simulink model "sl_groundvehicleDynamics"  (R2025b)
settings: Solver=ode45  StartTime=0.0  StopTime=2000  RelTol=1e-5  EnableMultiTasking=on
InitFcn:
  | mdl_robot;
values from neighbouring files (symbols this model uses):
  A = [1,0,0,dt,0,0;    0,1,0,0,dt,0;    0,0,1,0,0,dt;    0,0,0,1,0,0;    0,0,0,0,1,0;    0,0,0,0,0,1]    [kalman_init.m]    (also in mdl_robot.m = [ 1 0 0 Ts  0  0)
  B = [ Ts   0 ... (first row only)    [mdl_robot.m]
  C = eye(6)    [mdl_robot.m]
  D = zeros(6,2)    [mdl_robot.m]
  initial_state = [robot.X ; robot.Y; robot.Theta; 0; 0; 0]    [mdl_robot.m]
  optimized_waypoints = cuztomized_wp    [mdl_robot.m]
  R = Const_R .* eye(3)    [kalman_init.m]    (also in mdl_robot.m = 0.00316  * R)
undefined symbols (not defined in the file or in its folder): Discrete, obstacles, robot, Time
libraries: simulink x8, mobileRoboticsLib x6, simulink_extras x2, ctrlSharedLib x1, sharedTrackingLibrary x1
settings Model: Creator=sriramn  LastModifiedBy=minhn
settings SolverCC: ZeroCrossAlgorithm=Adaptive  AlgebraicLoopSolver=TrustRegion
settings DataIOCC: LimitDataPoints=on  SaveFormat=Array  ReturnWorkspaceOutputs=off
settings OptimizationCC: ReuseModelBlockBuffer=off  LifeSpan=inf
settings DebuggingCC: SolverPrmCheckMsg=warning  UnconnectedInputMsg=warning  UnconnectedOutputMsg=warning  UnconnectedLineMsg=warning  AllowSymbolicDim=off  SFUnexpectedBacktrackingDiag=warning  SFNoUnconditionalDefaultTransitionDiag=warning  SFExecutionAtInitializationDiag=none  ArithmeticOperatorsInVariantConditions=warning
settings HardwareCC: ProdBitPerPointer=32.0  ProdBitPerSizeT=32.0  ProdBitPerPtrDiffT=32.0  ProdLargestAtomicFloat=None  ProdIntDivRoundTo=Undefined  ProdEndianess=Unspecified  ProdWordSize=32.0  ProdHWDeviceType=32-bit Generic
settings ModelReferenceCC: EnableRefExpFcnMdlSchedulingChecks=on  ModelReferenceMinAlgLoopOccurrences=on  PropagateSignalLabelsOutOfModel=off
settings SFSimCC: SimUseLocalCustomCode=off  CustomCodeUndefinedFunction=UseInterfaceOnly
settings RTWCC: RTWUseLocalCustomCode=off  GPUComputeCapability=3.5
settings CodeAppCC: StateflowObjectComments=on
settings GRTTargetCC: TargetLangStandard=C89/C90 (ANSI)
settings ConfigComp: CovMetricSettings=dw  CovSaveCumulativeToWorkspaceVar=on  CovSaveSingleToWorkspaceVar=on  CovExternalEMLEnable=off  CovSFcnEnable=off
settings SimscapeCC: SimscapeNormalizeSystem=off  SimscapeLogDataHistory=5000  SimscapeLogDecimation=1
settings ConfigurationSet: Description=SimMechanics 2G
settings ExplorerConfigSet: InternalSimMechanicsExplorerSettings="<ExplorerConfiguration><canonicalview>planar_xy</canonicalview><AnimationSetting><BasePlaybackSpeed>1.0</BasePlaybackSpeed><PlaybackSpeedFactor>1.0</PlaybackSpeedFactor></AnimationSetting><TilePanel><TileInfo><Tiles Columns=\"1\" Count=\"1\" Rows=\"1\"><Column Left=\"2\" Weight=\"1\"/><Column Left=\"1628\"/><Row Top=\"2\" Weight=\"1\"/><Row Top=\"1072\"/><Tile Height=\"1\" Width=\"1\" X=\"0\" Y=\"0\"/></Tiles></TileInfo><SceneInfo><SceneViewer><BGColor><R>0.60000002384185791</R><G>0.60000002384185791</G><B>0.60000002384185791</B></BGColor><Camera><Position><X>0.22951840878551699</X><Y>0.32651610611526627</Y><Z>-0.27215421354393321</Z></Position><Center><X>-0.15775714411666431</X><Y>-0.15462825985839526</Y><Z>0.065702552916005602</Z></Center><Up><X>-0.56030137557930915</X><Y>0.72817587161684794</Y><Z>0.39474329445726858</Z></Up><Left>-0.21481383955700509</Left><Right>0.21481383955700509</Right><Bottom>-0.27569784609469139</Bottom><Top>0.27569784609469139</Top></Camera></SceneViewer></SceneInfo></TilePanel></ExplorerConfiguration>"

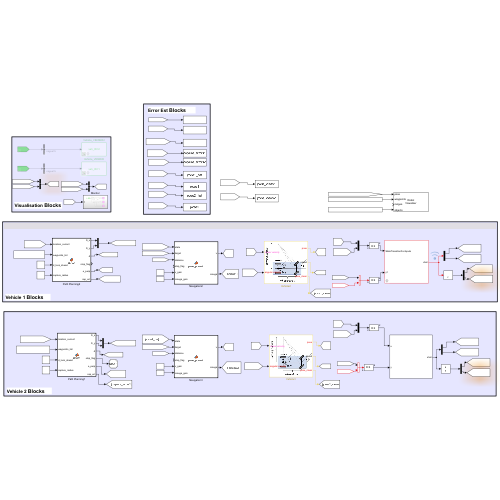
[thumbnail: Simulink's stored preview of the top-level diagram]
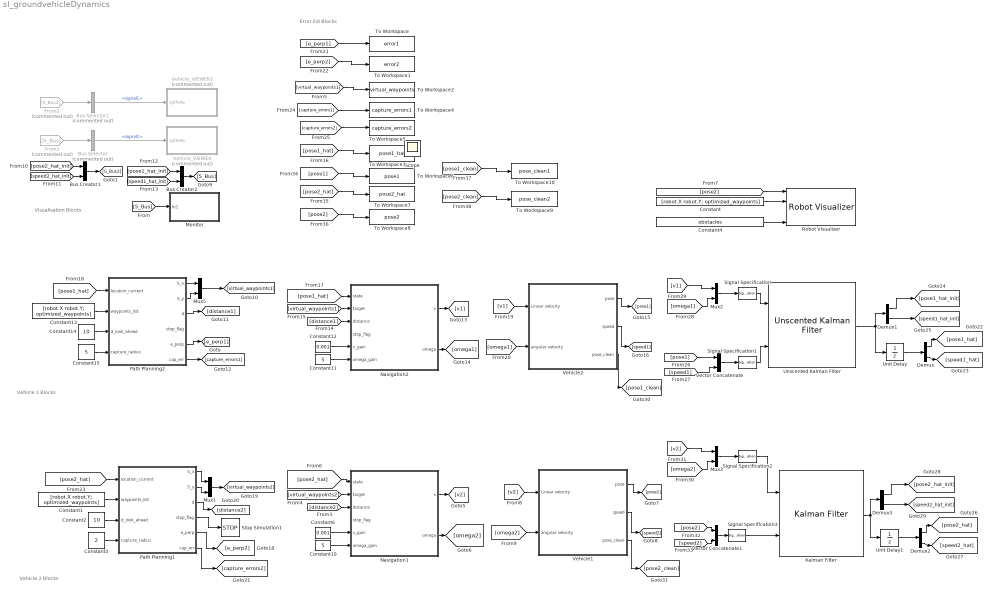
== system sl_groundvehicleDynamics ==
  note: Visualisation Blocks
  note: Vehicle 1 Blocks
  note: Vehicle 2 Blocks
  note: Error Est Blocks
  Bus Creator1 : BusCreator  Inputs=2
  Bus Creator2 : BusCreator  Inputs=2
  Bus Selector : BusSelector  Commented=on  OutputSignals=signal1
  Bus Selector1 : BusSelector  Commented=on  OutputSignals=signal1
  Constant : Constant  Value=[robot.X robot.Y; optimized_waypoints]
  Constant1 : Constant  Value=[robot.X robot.Y; optimized_waypoints]
  Constant10 : Constant  Value=5
  Constant11 : Constant  Value=5
  Constant12 : Constant  Value=0.001
  Constant13 : Constant  Value=[robot.X robot.Y; optimized_waypoints]
  Constant14 : Constant  Value=10
  Constant15 : Constant  Value=5
  Constant2 : Constant  Value=10
  Constant3 : Constant  Value=2
  Constant4 : Constant  Value=obstacles
  Constant6 : Constant  Value=0.001
  Demux{,1..3} (4 alike) : Demux  Outputs=2
  From1 : From  Commented=on  GotoTag=S_Bus
  From2 : From  Commented=on  GotoTag=S_Bus2
  Kalman Filter : ctrlSharedLib/Kalman Filter  TimeDomain=Discrete-Time  UseCurrentEstimator=on  ModelSource=Individual A, B, C, D matrices  ModelSourceVariable=ss(0.95,1,1,0,1)  A=A  B=B  C=C  D=D  NumberOfStates=6  NumberOfInputs=2  NumberOfOutputs=1  InitialEstimateSource=Dialog  X0=initial_state  P0=10  UseK=off  UseGH=off  NumberOfProcessNoiseInputs=1  G=1  TimeInvariantG=on  H=0  TimeInvariantH=on  Q=Q  TimeInvariantQ=on  R=R  TimeInvariantR=on  N=0  TimeInvariantN=on  AddInputPort=on  AddEnablePort=off  OutputEstimatedY=off  OutputP=off  Ts=-1
  Monitor : Subsystem
  Mux{1..3,5} (4 alike) : Mux  Inputs=2
  Navigation1 : MATLAB Function  TreatAsAtomicUnit=on
  Navigation2 : MATLAB Function  TreatAsAtomicUnit=on
  Path Planning1 : MATLAB Function  TreatAsAtomicUnit=on
  Path Planning2 : MATLAB Function  TreatAsAtomicUnit=on
  Robot Visualizer : mobileRoboticsLib/Environments/Robot Visualizer  robotRadius=0.25  mapName=map  showTrajectory=on  hasWaypoints=on  hasLidar=on  sensorOffset=[ 0, 0 ]  scanAngles=[ -pi/4, 0, pi/4 ]  hasObjDetector=on  objDetectorOffset=[ 0, 0 ]  objDetectorAngle=0  objDetectorFOV=pi/4  objDetectorMaxRange=5  objectColors=[ 1, 0, 0; 0, 1, 0; 0, 0, 1 ]  objectMarkers=s
  Signal Specification : SignalSpecification  Dimensions=2
  Signal Specification1 : SignalSpecification  Dimensions=6
  Signal Specification2 : SignalSpecification  Dimensions=2
  Signal Specification3 : SignalSpecification  Dimensions=6
  Stop Simulation1 : Stop
  To Workspace : ToWorkspace  VariableName=error1  SaveFormat=Timeseries  SampleTime=-1
  To Workspace1 : ToWorkspace  VariableName=error2  SaveFormat=Timeseries  SampleTime=-1
  To Workspace10 : ToWorkspace  VariableName=pose_clean1  SaveFormat=Timeseries  SampleTime=-1
  To Workspace2 : ToWorkspace  VariableName=virtual_waypoints  SaveFormat=Timeseries  SampleTime=-1
  To Workspace3 : ToWorkspace  VariableName=pose1_hat  SaveFormat=Timeseries  SampleTime=-1
  To Workspace4 : ToWorkspace  VariableName=capture_errors1  SaveFormat=Timeseries  SampleTime=-1
  To Workspace5 : ToWorkspace  VariableName=capture_errors2  SaveFormat=Timeseries  SampleTime=-1
  To Workspace6 : ToWorkspace  VariableName=pose1  SaveFormat=Timeseries  SampleTime=-1
  To Workspace7 : ToWorkspace  VariableName=pose2_hat  SaveFormat=Timeseries  SampleTime=-1
  To Workspace8 : ToWorkspace  VariableName=pose2  SaveFormat=Timeseries  SampleTime=-1
  To Workspace9 : ToWorkspace  VariableName=pose_clean2  SaveFormat=Timeseries  SampleTime=-1
  Unit Delay : UnitDelay  InitialCondition=[0;0;0;0;0;0]  SampleTime=-1  HasFrameUpgradeWarning=on
  Unit Delay1 : UnitDelay  InitialCondition=[0;0;0;0;0;0]  SampleTime=-1  HasFrameUpgradeWarning=on
  Unscented Kalman Filter : sharedTrackingLibrary/Unscented Kalman Filter  StateTransitionFcn=fState  HasAdditiveProcessNoise=Additive  ProcessNoise=Q  HasTimeVaryingProcessNoise=off  HasStateTransitionFcnExtraArgument=1  InitialState=initial_state  InitialStateCovariance=P0  Alpha=Alpha  Beta=2  Kappa=0  MeasurementFcn1=hMeas  HasMeasurementEnablePort1=off  HasAdditiveMeasurementNoise1=Additive  MeasurementNoise1=R  HasTimeVaryingMeasurementNoise1=off  HasMeasurementFcnExtraArgument1=0  HasMeasurementWrapping1=on  MeasurementFcn2=myMeasurementFcn  HasMeasurementEnablePort2=off  HasAdditiveMeasurementNoise2=Additive  MeasurementNoise2=1  HasTimeVaryingMeasurementNoise2=off  HasMeasurementFcnExtraArgument2=0  HasMeasurementWrapping2=off  MeasurementFcn3=myMeasurementFcn  HasMeasurementEnablePort3=off  HasAdditiveMeasurementNoise3=Additive  MeasurementNoise3=1  HasTimeVaryingMeasurementNoise3=off  HasMeasurementFcnExtraArgument3=0  HasMeasurementWrapping3=off  MeasurementFcn4=myMeasurementFcn  HasMeasurementEnablePort4=off  HasAdditiveMeasurementNoise4=Additive  MeasurementNoise4=1  HasTimeVaryingMeasurementNoise4=off  HasMeasurementFcnExtraArgument4=0  HasMeasurementWrapping4=off  MeasurementFcn5=myMeasurementFcn  HasMeasurementEnablePort5=off  HasAdditiveMeasurementNoise5=Additive  MeasurementNoise5=1  HasTimeVaryingMeasurementNoise5=off  HasMeasurementFcnExtraArgument5=0  HasMeasurementWrapping5=off  EnableMultirate=off  StateTransitionFcnSampleTime=1  MeasurementFcn1SampleTime=1  MeasurementFcn2SampleTime=1  MeasurementFcn3SampleTime=1  MeasurementFcn4SampleTime=1  MeasurementFcn5SampleTime=1  UseCurrentEstimator=on  OutputStateCovariance=off  DataType=double  SampleTime=0.05  NumberOfMeasurements=1
      settings: LibrarySourceBlock=cstblocks/State Estimation/Unscented Kalman Filter
  Vector Concatenate : Concatenate
  Vector Concatenate1 : Concatenate
  Vehicle1 : Subsystem
      mask Display: image('vehicle.jpg');
  Vehicle2 : Subsystem
      mask Display: image('vehicle.jpg');
  Vehicle_VIEWER : Subsystem  Commented=on  mask{wp_mat=optimized_waypoints, veh_ID_num=1, veh_init_xytheta=[robot.X robot.Y robot.Theta], Ts=0.5}
      mask prompts: wp_mat "Waypoint matrix for arena [x_col, y_col] (m)"; veh_ID_num "Vehicle ID number"; veh_init_xytheta "Initial pose [x,y,theta]"; Ts "Sample time for updating animation (secs)"
      mask TypeOptions veh_ID_num: 1 | 2 | 3 | 4
      mask DialogControl Control2 Prompt: Animate simulation of Differential Drive Robot (DDR)
      mask Display: fprintf('veh_ID=%d',veh_ID_num);
  Vehicle_VIEWER2 : Subsystem  Commented=on  mask{wp_mat=optimized_waypoints, veh_ID_num=2, veh_init_xytheta=[robot.X robot.Y robot.Theta], Ts=0.5}
      mask prompts: wp_mat "Waypoint matrix for arena [x_col, y_col] (m)"; veh_ID_num "Vehicle ID number"; veh_init_xytheta "Initial pose [x,y,theta]"; Ts "Sample time for updating animation (secs)"
      mask TypeOptions veh_ID_num: 1 | 2 | 3 | 4
      mask DialogControl Control2 Prompt: Animate simulation of Differential Drive Robot (DDR)
      mask Display: fprintf('veh_ID=%d',veh_ID_num);
  Scope : Scope
      settings: ActiveDisplayYMinimum=0.07  ActiveDisplayYMaximum=0.09
  wires:
  Constant6/1 -> Navigation1/5(v_gain)
  Vehicle1/1(pose) -> [pose2]
  Constant10/1 -> Navigation1/6(omega_gain)
  [distance2] -> Navigation1/3(distance)
  [virtual_waypoints2] -> Navigation1/2(target)
  Navigation1/1(v) -> [v2]
  [pose2_hat] -> Navigation1/1(state)
  Vehicle1/2(speed) -> [speed2]
  [v2] -> Vehicle1/1(Linear velocity)
  [omega2] -> Vehicle1/2(angular velocity)
  [pose1_hat_init] -> Bus Creator2/1
  Bus Creator2/1 -> [S_Bus]
  [speed1_hat_init] -> Bus Creator2/2
  Bus Creator1/1 -> [S_Bus2]
  [pose2_hat_init] -> Bus Creator1/1
  From2/1 -> Bus Selector1/1
  [speed2_hat_init] -> Bus Creator1/2
  [S_Bus] -> Monitor/1(In1)
  Bus Selector1/1 -> Vehicle_VIEWER2/1(xytheta)  "<signal1>"
  Bus Selector/1 -> Vehicle_VIEWER/1(xytheta)  "<signal1>"
  From1/1 -> Bus Selector/1
  Constant14/1 -> Path Planning2/3(d_look_ahead)
  Navigation2/2(omega) -> [omega1]
  Constant15/1 -> Path Planning2/4(capture_radius)
  Vehicle2/1(pose) -> [pose1]
  Path Planning2/1(S_x) -> Mux5/1
  Mux5/1 -> [virtual_waypoints1]
  [pose1_hat] -> Path Planning2/1(location_current)
  Constant11/1 -> Navigation2/6(omega_gain)
  Constant13/1 -> Path Planning2/2(waypoints_list)
  Path Planning2/2(S_y) -> Mux5/2
  [distance1] -> Navigation2/3(distance)
  [v1] -> Vehicle2/1(Linear velocity)
  Constant12/1 -> Navigation2/5(v_gain)
  [omega1] -> Vehicle2/2(angular velocity)
  Path Planning2/3(d) -> [distance1]
  [pose1_hat] -> Navigation2/1(state)
  [virtual_waypoints1] -> Navigation2/2(target)
  Vehicle2/2(speed) -> [speed1]
  Navigation2/1(v) -> [v1]
  Path Planning2/5(e_perp) -> [e_perp1]
  [e_perp2] -> To Workspace1/1
  [pose2_hat] -> Path Planning1/1(location_current)
  Constant2/1 -> Path Planning1/3(d_look_ahead)
  Path Planning1/5(e_perp) -> [e_perp2]
  Path Planning1/3(d) -> [distance2]
  Constant1/1 -> Path Planning1/2(waypoints_list)
  Constant3/1 -> Path Planning1/4(capture_radius)
  Path Planning1/2(S_y) -> Mux1/2
  Mux1/1 -> [virtual_waypoints2]
  Path Planning1/1(S_x) -> Mux1/1
  [e_perp1] -> To Workspace/1
  [virtual_waypoints1] -> To Workspace2/1
  [pose1_hat] -> To Workspace3/1
  Path Planning2/6(cap_err) -> [capture_errors1]
  [capture_errors1] -> To Workspace4/1
  Path Planning1/6(cap_err) -> [capture_errors2]
  [capture_errors2] -> To Workspace5/1
  Mux2/1 -> Signal Specification/1
  [omega1] -> Mux2/2
  Demux/1 -> [pose1_hat]
  Signal Specification/1 -> Unscented Kalman Filter/1
  Unscented Kalman Filter/1 -> Unit Delay/1, Demux1/1
  Signal Specification1/1 -> Unscented Kalman Filter/2
  [v1] -> Mux2/1
  Demux/2 -> [speed1_hat]
  Unit Delay/1 -> Demux/1
  [pose1] -> Vector Concatenate/1
  Demux1/2 -> [speed1_hat_init]
  Demux1/1 -> [pose1_hat_init]
  [speed1] -> Vector Concatenate/2
  Vector Concatenate/1 -> Signal Specification1/1
  [v2] -> Mux3/1
  Signal Specification2/1 -> Kalman Filter/1
  [omega2] -> Mux3/2
  Mux3/1 -> Signal Specification2/1
  Vector Concatenate1/1 -> Signal Specification3/1
  [speed2] -> Vector Concatenate1/2
  [pose2] -> Vector Concatenate1/1
  Signal Specification3/1 -> Kalman Filter/2
  Demux3/1 -> [pose2_hat_init]
  Unit Delay1/1 -> Demux2/1
  Kalman Filter/1 -> Demux3/1, Unit Delay1/1
  Demux2/1 -> [pose2_hat]
  Demux2/2 -> [speed2_hat]
  Demux3/2 -> [speed2_hat_init]
  Navigation1/2(omega) -> [omega2]
  [pose1] -> To Workspace6/1
  [pose2_hat] -> To Workspace7/1
  [pose2] -> To Workspace8/1
  [pose1_clean] -> To Workspace10/1
  Vehicle2/3(pose_clean) -> [pose1_clean]
  [pose2_clean] -> To Workspace9/1
  Vehicle1/3(pose_clean) -> [pose2_clean]
  Path Planning1/4(stop_flag) -> Stop Simulation1/1
  Constant/1 -> Robot Visualizer/2
  [pose2] -> Robot Visualizer/1
  Constant4/1 -> Robot Visualizer/4

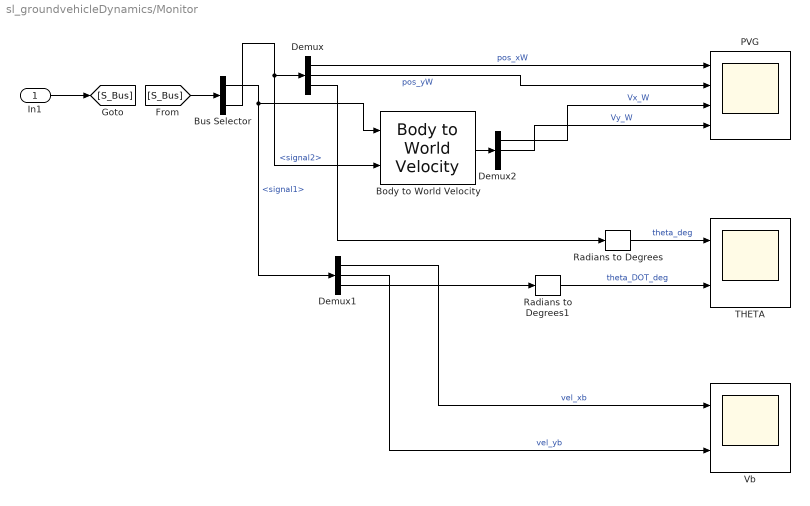
== system sl_groundvehicleDynamics/Monitor ==
  In1 : Inport
  Body to World Velocity : mobileRoboticsLib/Utilities/Body to World Velocity
      settings: SourceProductName=Mobile Robotics Simulation Toolbox
  Bus Selector : BusSelector  OutputSignals=signal1,signal2
  Demux : Demux  Outputs=3
  Demux1 : Demux  Outputs=3
  Demux2 : Demux  Outputs=3
  PVG : Scope  NumInputPorts=4
      settings: ActiveDisplayYMinimum=-3.02358  ActiveDisplayYMaximum=27.35477
  Radians to Degrees : simulink_extras/Transformations/Radians to Degrees
  Radians to Degrees1 : simulink_extras/Transformations/Radians to Degrees
  THETA : Scope  NumInputPorts=2
      settings: ActiveDisplayYMinimum=-8.72937  ActiveDisplayYMaximum=60.06611  DataLoggingVariableName=ScopeData2
  Vb : Scope  NumInputPorts=2
      settings: ActiveDisplayYMinimum=0.05577  ActiveDisplayYMaximum=0.8929
  wires:
  In1/1 -> [S_Bus]
  [S_Bus] -> Bus Selector/1
  Demux/1 -> PVG/1  "pos_xW"
  Demux/2 -> PVG/2  "pos_yW"
  Radians to Degrees1/1 -> THETA/2  "theta_DOT_deg"
  Radians to Degrees/1 -> THETA/1  "theta_deg"
  Demux1/3 -> Radians to Degrees1/1
  Demux/3 -> Radians to Degrees/1
  Bus Selector/1 -> Demux1/1, Body to World Velocity/1  "<signal1>"
  Body to World Velocity/1 -> Demux2/1
  Demux2/1 -> PVG/3  "Vx_W"
  Demux2/2 -> PVG/4  "Vy_W"
  Demux1/1 -> Vb/1  "vel_xb"
  Demux1/2 -> Vb/2  "vel_yb"
  Bus Selector/2 -> Body to World Velocity/2, Demux/1  "<signal2>"

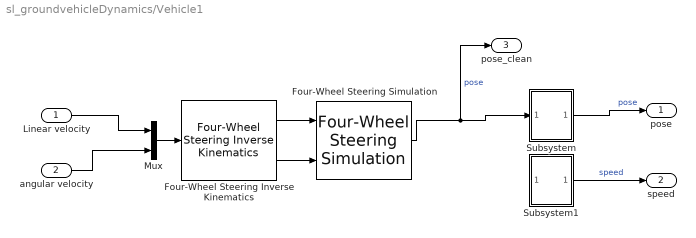
== system sl_groundvehicleDynamics/Vehicle1 ==
  Linear velocity : Inport
  angular velocity : Inport  Port=2
  Four-Wheel Steering Inverse Kinematics : mobileRoboticsLib/Kinematic Models/Four-Wheel Steering/Four-Wheel Steering Inverse Kinematics  wheelRadius=0.1  frontWheelDist=0.25  rearWheelDist=0.25  ikMode=Front Steering
      settings: SourceProductName=Mobile Robotics Simulation Toolbox
  Four-Wheel Steering Simulation : mobileRoboticsLib/Kinematic Models/Four-Wheel Steering/Four-Wheel Steering Simulation  wheelRadius=0.1  frontWheelDist=0.25  rearWheelDist=0.25  initX=robot.X  initY=robot.Y  initAngle=robot.Theta  Ts=0.05
      settings: SourceProductName=Mobile Robotics Simulation Toolbox
  Mux : Mux  Inputs=2
  Subsystem : Subsystem
  Subsystem1 : Subsystem
  pose : Outport  VectorParamsAs1DForOutWhenUnconnected=off
  speed : Outport  Port=2
  pose_clean : Outport  Port=3  VectorParamsAs1DForOutWhenUnconnected=off
  wires:
  angular velocity/1 -> Mux/2
  Linear velocity/1 -> Mux/1
  Mux/1 -> Four-Wheel Steering Inverse Kinematics/1
  Four-Wheel Steering Simulation/1 -> pose_clean/1, Subsystem/1(In1)  "pose"
  ? -> Subsystem1/1(In1)  "speed"
  Four-Wheel Steering Inverse Kinematics/1 -> Four-Wheel Steering Simulation/1
  Four-Wheel Steering Inverse Kinematics/2 -> Four-Wheel Steering Simulation/2
  Subsystem/1(pose) -> pose/1  "pose"
  Subsystem1/1(speed) -> speed/1  "speed"

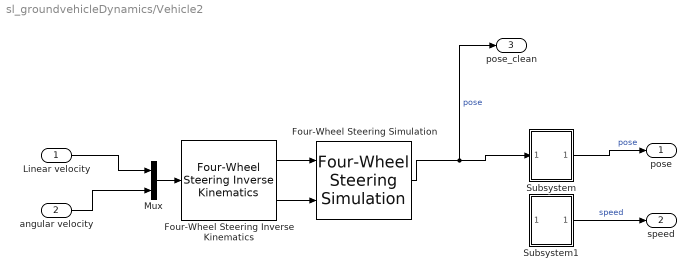
== system sl_groundvehicleDynamics/Vehicle2 ==
  Linear velocity : Inport
  angular velocity : Inport  Port=2
  Four-Wheel Steering Inverse Kinematics : mobileRoboticsLib/Kinematic Models/Four-Wheel Steering/Four-Wheel Steering Inverse Kinematics  wheelRadius=0.1  frontWheelDist=0.25  rearWheelDist=0.25  ikMode=Front Steering
      settings: SourceProductName=Mobile Robotics Simulation Toolbox
  Four-Wheel Steering Simulation : mobileRoboticsLib/Kinematic Models/Four-Wheel Steering/Four-Wheel Steering Simulation  wheelRadius=0.1  frontWheelDist=0.25  rearWheelDist=0.25  initX=robot.X  initY=robot.Y  initAngle=robot.Theta  Ts=0.05
      settings: SourceProductName=Mobile Robotics Simulation Toolbox
  Mux : Mux  Inputs=2
  Subsystem : Subsystem
  Subsystem1 : Subsystem
  pose : Outport  VectorParamsAs1DForOutWhenUnconnected=off
  speed : Outport  Port=2
  pose_clean : Outport  Port=3  VectorParamsAs1DForOutWhenUnconnected=off
  wires:
  angular velocity/1 -> Mux/2
  Linear velocity/1 -> Mux/1
  Mux/1 -> Four-Wheel Steering Inverse Kinematics/1
  Four-Wheel Steering Simulation/1 -> pose_clean/1, Subsystem/1(In1)  "pose"
  Four-Wheel Steering Inverse Kinematics/1 -> Four-Wheel Steering Simulation/1
  Four-Wheel Steering Inverse Kinematics/2 -> Four-Wheel Steering Simulation/2
  Subsystem/1(pose) -> pose/1  "pose"
  Subsystem1/1(speed) -> speed/1  "speed"
  ? -> Subsystem1/1(In1)

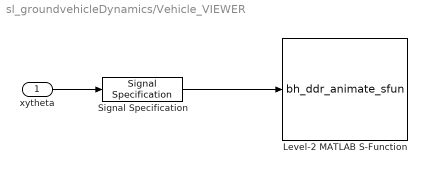
== system sl_groundvehicleDynamics/Vehicle_VIEWER ==
  xytheta : Inport
  Level-2 MATLAB S-Function : M-S-Function  FunctionName=bh_ddr_animate_sfun  Parameters=Ts, wp_mat, veh_ID_num, veh_init_xytheta
  Signal Specification : SignalSpecification  Dimensions=3
  wires:
  xytheta/1 -> Signal Specification/1
  Signal Specification/1 -> Level-2 MATLAB S-Function/1

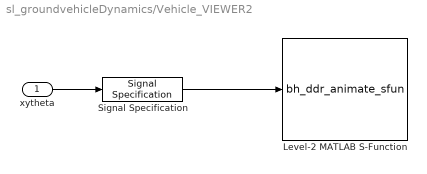
== system sl_groundvehicleDynamics/Vehicle_VIEWER2 ==
  xytheta : Inport
  Level-2 MATLAB S-Function : M-S-Function  FunctionName=bh_ddr_animate_sfun  Parameters=Ts, wp_mat, veh_ID_num, veh_init_xytheta
  Signal Specification : SignalSpecification  Dimensions=3
  wires:
  xytheta/1 -> Signal Specification/1
  Signal Specification/1 -> Level-2 MATLAB S-Function/1

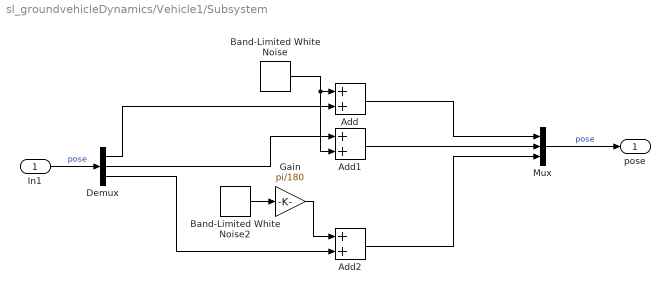
== system sl_groundvehicleDynamics/Vehicle1/Subsystem ==
  In1 : Inport
  Add : Sum
  Add1 : Sum
  Add2 : Sum
  Band-Limited White Noise : simulink/Sources/Band-Limited White Noise  Cov=[0.001]  Ts=0.1  seed=[23341]
  Band-Limited White Noise2 : simulink/Sources/Band-Limited White Noise  Cov=[0.41]  Ts=0.1  seed=[23341]
  Demux : Demux  Outputs=3
  Gain : Gain  Gain=pi/180
  Mux : Mux  Inputs=3
  pose : Outport
  wires:
  Add1/1 -> Mux/2
  Add2/1 -> Mux/3
  Demux/2 -> Add1/1
  Band-Limited White Noise2/1 -> Gain/1
  Demux/3 -> Add2/2
  Band-Limited White Noise/1 -> Add1/2, Add/1
  In1/1 -> Demux/1  "pose"
  Demux/1 -> Add/2
  Gain/1 -> Add2/1
  Mux/1 -> pose/1  "pose"
  Add/1 -> Mux/1

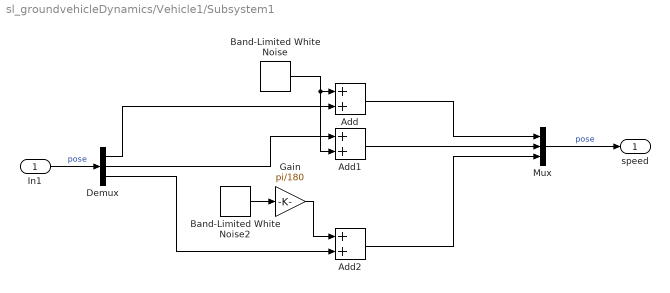
== system sl_groundvehicleDynamics/Vehicle1/Subsystem1 ==
  In1 : Inport
  Add : Sum
  Add1 : Sum
  Add2 : Sum
  Band-Limited White Noise : simulink/Sources/Band-Limited White Noise  Cov=[0.001]  Ts=0.1  seed=[23341]
  Band-Limited White Noise2 : simulink/Sources/Band-Limited White Noise  Cov=[0.41]  Ts=0.1  seed=[23341]
  Demux : Demux  Outputs=3
  Gain : Gain  Gain=pi/180
  Mux : Mux  Inputs=3
  speed : Outport
  wires:
  Add1/1 -> Mux/2
  Add2/1 -> Mux/3
  Demux/2 -> Add1/1
  Band-Limited White Noise2/1 -> Gain/1
  Demux/3 -> Add2/2
  Band-Limited White Noise/1 -> Add1/2, Add/1
  In1/1 -> Demux/1  "pose"
  Demux/1 -> Add/2
  Gain/1 -> Add2/1
  Mux/1 -> speed/1  "pose"
  Add/1 -> Mux/1

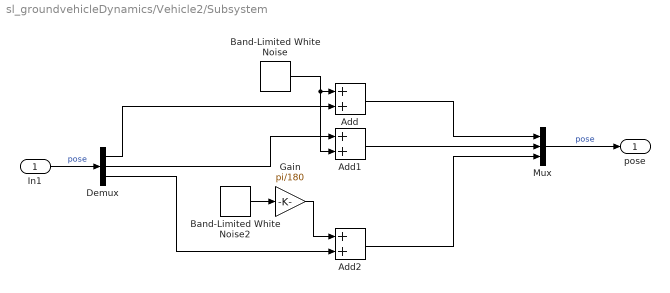
== system sl_groundvehicleDynamics/Vehicle2/Subsystem ==
  In1 : Inport
  Add : Sum
  Add1 : Sum
  Add2 : Sum
  Band-Limited White Noise : simulink/Sources/Band-Limited White Noise  Cov=[0.001]  Ts=0.1  seed=[23341]
  Band-Limited White Noise2 : simulink/Sources/Band-Limited White Noise  Cov=[0.41]  Ts=0.1  seed=[23341]
  Demux : Demux  Outputs=3
  Gain : Gain  Gain=pi/180
  Mux : Mux  Inputs=3
  pose : Outport
  wires:
  Add1/1 -> Mux/2
  Add2/1 -> Mux/3
  Demux/2 -> Add1/1
  Band-Limited White Noise2/1 -> Gain/1
  Demux/3 -> Add2/2
  Band-Limited White Noise/1 -> Add1/2, Add/1
  In1/1 -> Demux/1  "pose"
  Demux/1 -> Add/2
  Gain/1 -> Add2/1
  Mux/1 -> pose/1  "pose"
  Add/1 -> Mux/1

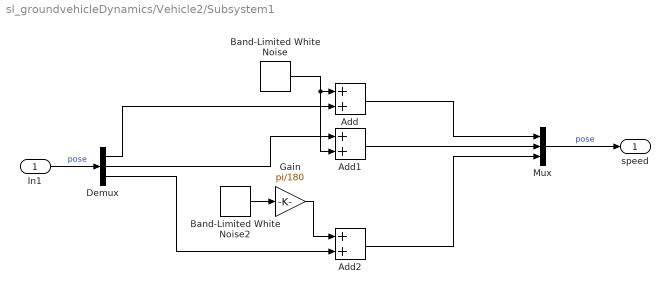
== system sl_groundvehicleDynamics/Vehicle2/Subsystem1 ==
  In1 : Inport
  Add : Sum
  Add1 : Sum
  Add2 : Sum
  Band-Limited White Noise : simulink/Sources/Band-Limited White Noise  Cov=[0.001]  Ts=0.1  seed=[23341]
  Band-Limited White Noise2 : simulink/Sources/Band-Limited White Noise  Cov=[0.41]  Ts=0.1  seed=[23341]
  Demux : Demux  Outputs=3
  Gain : Gain  Gain=pi/180
  Mux : Mux  Inputs=3
  speed : Outport
  wires:
  Add1/1 -> Mux/2
  Add2/1 -> Mux/3
  Demux/2 -> Add1/1
  Band-Limited White Noise2/1 -> Gain/1
  Demux/3 -> Add2/2
  Band-Limited White Noise/1 -> Add1/2, Add/1
  In1/1 -> Demux/1  "pose"
  Demux/1 -> Add/2
  Gain/1 -> Add2/1
  Mux/1 -> speed/1  "pose"
  Add/1 -> Mux/1

== matlab function sl_groundvehicleDynamics/Path Planning1 ==
  data: location_current input size=3; S_x output; waypoints_list input; d_look_ahead input; S_y output; d output; stop_flag output; capture_radius input; e_perp output; cap_err output
function [S_x, S_y, d, stop_flag, e_perp, cap_err] = RVW(location_current, waypoints_list, d_look_ahead , capture_radius)
% RVWP computes the Rear-View Waypoint (RVWP) for path following
% and cross-track error for plotting
% Modified for Simulink compatibility: returns latest capture error only.

xd = waypoints_list(:,1);
yd = waypoints_list(:,2);

x = location_current(1);
y = location_current(2);

% Persistent variable to remember current waypoint index
persistent n
if isempty(n)
    n = 1;  % Start from the first waypoint
end

stop_flag = 0;
e_perp = 0;      % default
cap_err  = NaN;  % default: no capture at this step

% Distance to next waypoint
if n < length(xd)
    stop_flag = 0;
    d = sqrt((x - xd(n+1))^2 + (y - yd(n+1))^2);

    % Distance & angles for RVWP
    Ru = sqrt((xd(n) - x)^2 + (yd(n) - y)^2);
    theta = atan2(yd(min(n+1,end)) - yd(n), xd(min(n+1,end)) - xd(n));
    theta_u = atan2(y - yd(n), x - xd(n));
    beta = theta - theta_u;
    R = Ru * cos(beta);

    % Compute RVWP
    S_x = xd(n) + (R + d_look_ahead)*cos(theta);
    S_y = yd(n) + (R + d_look_ahead)*sin(theta);

    % Cross-track error (perpendicular to path segment)
    vec_path = [xd(n+1)-xd(n), yd(n+1)-yd(n)];
    vec_to_vehicle = [x - xd(n), y - yd(n)];
    R_path = dot(vec_to_vehicle, vec_path)/norm(vec_path);  % along-track
    e_perp = sqrt(max(0, norm(vec_to_vehicle)^2 - R_path^2)); % perpendicular

    % Waypoint capture check
    if d < capture_radius
        cap_err = d;   % capture error at this waypoint
        n = n + 1;     % Move to next waypoint
    end
else
    % Last waypoint
    d = sqrt((x - xd(n))^2 + (y - yd(n))^2);
    S_x = xd(n);
    S_y = yd(n);
    e_perp = sqrt((x - xd(n))^2 + (y - yd(n))^2);  % distance to final waypoint
    if d < 1
        stop_flag = 1;
        cap_err = d;  % final capture error
    end
end

end

== matlab function sl_groundvehicleDynamics/Navigation1 ==
  data: state input; v output; omega output; target input; distance input; stop_flag input; v_gain input; omega_gain input
function [v, omega] = pure_pursuit(state, target, distance, stop_flag, v_gain, omega_gain)
%PURE_PURSUIT Compute linear and angular velocity using pure pursuit
%   state: [x, y, theta]
%   target: [x_target, y_target]
%   distance: distance to target
%   stop_flag: 0 = move, 1 = stop



% Linear velocity (minimum 0.5 m/s)
v = distance * v_gain;  % Proportional Control
v = max(v, 2);
%v =30;
% Relative position
dx = target(1) - state(1);
dy = target(2) - state(2);

% Line-of-sight angle
gamma = atan2(dy, dx);

% Robot orientation
theta = state(3);

% Pure pursuit angular velocity
omega = omega_gain * angdiff(theta, gamma);
if stop_flag == 1
    v = 0;
    omega = 0;
    return;
end
end

== matlab function sl_groundvehicleDynamics/Navigation2 ==
  data: state input; v output; omega output; target input; distance input; stop_flag input; v_gain input; omega_gain input
function [v, omega] = pure_pursuit(state, target, distance, stop_flag, v_gain, omega_gain)
%PURE_PURSUIT Compute linear and angular velocity using pure pursuit
%   state: [x, y, theta]
%   target: [x_target, y_target]
%   distance: distance to target
%   stop_flag: 0 = move, 1 = stop



% Linear velocity (minimum 0.5 m/s)
v = distance * v_gain;  % Proportional Control
v = max(v, 20);
%v = 30;
% Relative position
dx = target(1) - state(1);
dy = target(2) - state(2);

% Line-of-sight angle
gamma = atan2(dy, dx);

% Robot orientation
theta = state(3);

% Pure pursuit angular velocity
omega = omega_gain * angdiff(theta, gamma);
if stop_flag == 1
    v = 0;
    omega = 0;
    return;
end
end

== matlab function sl_groundvehicleDynamics/Path Planning2 ==
  data: location_current input; S_x output; waypoints_list input; d_look_ahead input; S_y output; d output; stop_flag output; capture_radius input; e_perp output; cap_err output
function [S_x, S_y, d, stop_flag, e_perp, cap_err] = RVW(location_current, waypoints_list, d_look_ahead , capture_radius)
% RVWP computes the Rear-View Waypoint (RVWP) for path following
% and cross-track error for plotting
% Modified for Simulink compatibility: returns latest capture error only.

xd = waypoints_list(:,1);
yd = waypoints_list(:,2);

x = location_current(1);
y = location_current(2);

% Persistent variable to remember current waypoint index
persistent n
if isempty(n)
    n = 1;  % Start from the first waypoint
end

stop_flag = 0;
e_perp = 0;      % default
cap_err  = NaN;  % default: no capture at this step

% Distance to next waypoint
if n < length(xd)
    stop_flag = 0;
    d = sqrt((x - xd(n+1))^2 + (y - yd(n+1))^2);

    % Distance & angles for RVWP
    Ru = sqrt((xd(n) - x)^2 + (yd(n) - y)^2);
    theta = atan2(yd(min(n+1,end)) - yd(n), xd(min(n+1,end)) - xd(n));
    theta_u = atan2(y - yd(n), x - xd(n));
    beta = theta - theta_u;
    R = Ru * cos(beta);

    % Compute RVWP
    S_x = xd(n) + (R + d_look_ahead)*cos(theta);
    S_y = yd(n) + (R + d_look_ahead)*sin(theta);

    % Cross-track error (perpendicular to path segment)
    vec_path = [xd(n+1)-xd(n), yd(n+1)-yd(n)];
    vec_to_vehicle = [x - xd(n), y - yd(n)];
    R_path = dot(vec_to_vehicle, vec_path)/norm(vec_path);  % along-track
    e_perp = sqrt(max(0, norm(vec_to_vehicle)^2 - R_path^2)); % perpendicular

    % Waypoint capture check
    if d < capture_radius
        cap_err = d;   % capture error at this waypoint
        n = n + 1;     % Move to next waypoint
    end
else
    % Last waypoint
    d = sqrt((x - xd(n))^2 + (y - yd(n))^2);
    S_x = xd(n);
    S_y = yd(n);
    e_perp = sqrt((x - xd(n))^2 + (y - yd(n))^2);  % distance to final waypoint
    if d < 1
        stop_flag = 1;
        cap_err = d;  % final capture error
    end
end

end
